simulink model "cv2simu"  (R2020a)
settings: Solver=VariableStepAuto  StartTime=0.0  StopTime=2  RelTol=1e-3
values from neighbouring files (symbols this model uses):
  A = [   0    1 ... (first row only)    [cv2.m]
  b = 100    [cv2.m]
  B = [0; 1/m]    [cv2.m]
  C = [1 ,0]    [cv2.m]
  D = 0    [cv2.m]
  discreteStateSpace = c2d(stateSpace, 0.0001)    [cv2.m]
  k = 10000    [cv2.m]
  m = 10    [cv2.m]
libraries: cstblocks x1
settings Model: Creator=Ondra  LastModifiedBy=Ondra
settings DataIOCC: Refine=100

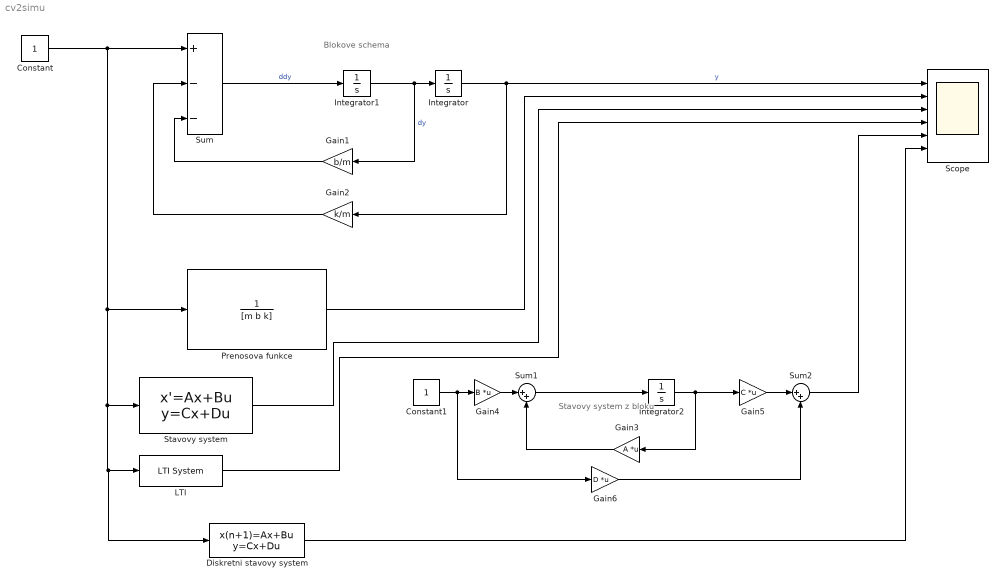
== system cv2simu ==
  note: Blokove schema
  note: Stavovy system z bloku
  Constant : Constant
  Constant1 : Constant
  Diskretni stavovy system : DiscreteStateSpace  A=discreteStateSpace.A  B=discreteStateSpace.B  C=discreteStateSpace.C  D=discreteStateSpace.D  SampleTime=-1
  Gain1 : Gain  Gain=b/m
  Gain2 : Gain  Gain=k/m
  Gain3 : Gain  Gain=A  Multiplication=Matrix(K*u)
  Gain4 : Gain  Gain=B  Multiplication=Matrix(K*u)
  Gain5 : Gain  Gain=C  Multiplication=Matrix(K*u)
  Gain6 : Gain  Gain=D  Multiplication=Matrix(K*u)
  Integrator : Integrator
  Integrator1 : Integrator
  Integrator2 : Integrator
  LTI : cstblocks/LTI System  sys=tf(1,[m b k])  IC=[]
  Prenosova funkce : TransferFcn  Denominator=[m b k]
  Scope : Scope  NumInputPorts=6
  Stavovy system : StateSpace  A=A  B=B  C=C  D=D  InitialCondition=0
  Sum : Sum  Inputs=+--
  Sum1 : Sum  Inputs=|++
  Sum2 : Sum  Inputs=|++
  wires:
  Integrator1/1 -> Gain1/1, Integrator/1  "dy"
  Integrator/1 -> Gain2/1, Scope/1  "y"
  Sum/1 -> Integrator1/1  "ddy"
  Constant/1 -> Diskretni stavovy system/1, LTI/1, Stavovy system/1, Prenosova funkce/1, Sum/1
  Gain1/1 -> Sum/3
  Gain2/1 -> Sum/2
  Prenosova funkce/1 -> Scope/2
  Sum1/1 -> Integrator2/1
  Constant1/1 -> Gain6/1, Gain4/1
  Gain4/1 -> Sum1/1
  Integrator2/1 -> Gain5/1, Gain3/1
  Stavovy system/1 -> Scope/3
  LTI/1 -> Scope/4
  Gain6/1 -> Sum2/2
  Gain5/1 -> Sum2/1
  Sum2/1 -> Scope/5
  Diskretni stavovy system/1 -> Scope/6
  Gain3/1 -> Sum1/2
